simulink model "QuarterCarSim"  (R2026a)
settings: Solver=ode45  StopTime=5  RelTol=1e-8
undefined symbols (not defined in the file or in its folder): Amp, b_s, b_u, k_s, k_u, m_s, m_u, omega
settings Model: Creator=tyres  LastModifiedBy=tyres

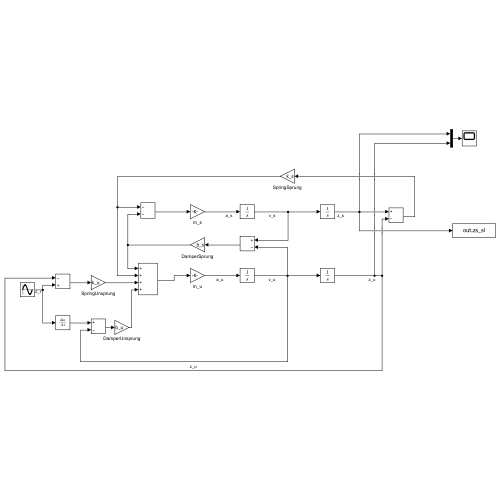
[thumbnail: Simulink's stored preview of the top-level diagram]
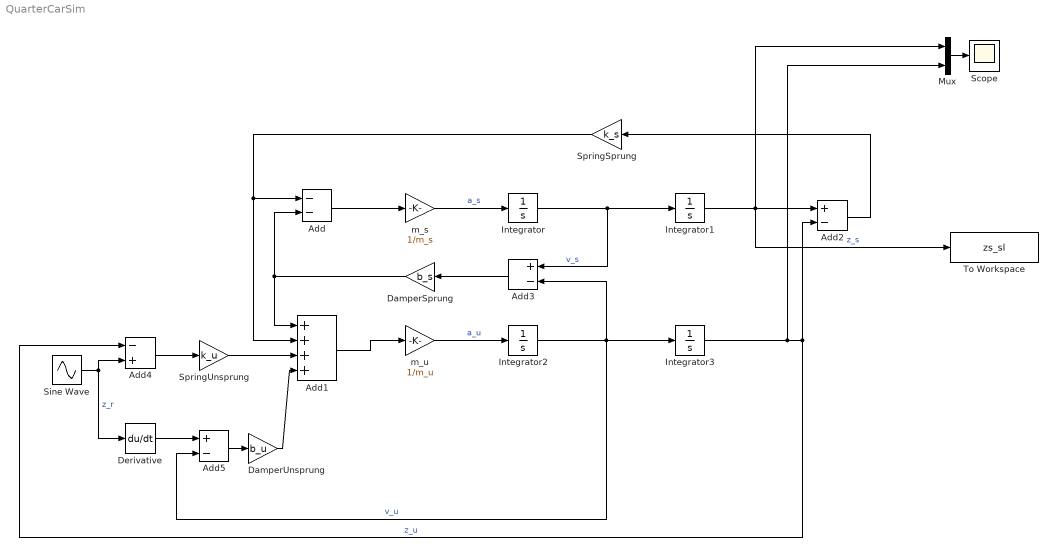
== system QuarterCarSim ==
  Add : Sum  Inputs=--
  Add1 : Sum  Inputs=++++
  Add2 : Sum  Inputs=+-
  Add3 : Sum  Inputs=+-
  Add4 : Sum  Inputs=-+
  Add5 : Sum  Inputs=+-
  DamperSprung : Gain  Gain=b_s
  DamperUnsprung : Gain  Gain=b_u
  Derivative : Derivative
  Integrator{,1..3} (4 alike) : Integrator
  Mux : Mux  Inputs=2
  Scope : Scope
      settings: ActiveDisplayYMinimum=-0.0072983920205625117  ActiveDisplayYMaximum=0.0069875189139344419
  Sine Wave : Sin  Amplitude=Amp  Frequency=omega  SampleTime=0
  SpringSprung : Gain  Gain=k_s
  SpringUnsprung : Gain  Gain=k_u
  To Workspace : ToWorkspace  VariableName=zs_sl  SaveFormat=Timeseries  SampleTime=-1
  m_s : Gain  Gain=1/m_s
  m_u : Gain  Gain=1/m_u
  wires:
  Integrator/1 -> Add3/1, Integrator1/1  "v_s"
  Integrator2/1 -> Add5/2, Add3/2, Integrator3/1  "v_u"
  m_s/1 -> Integrator/1  "a_s"
  Integrator3/1 -> Mux/2, Add4/1, Add2/2  "z_u"
  m_u/1 -> Integrator2/1  "a_u"
  Add1/1 -> m_u/1
  Add/1 -> m_s/1
  Integrator1/1 -> To Workspace/1, Mux/1, Add2/1  "z_s"
  Add2/1 -> SpringSprung/1
  SpringSprung/1 -> Add/1, Add1/2
  Add3/1 -> DamperSprung/1
  DamperSprung/1 -> Add1/1, Add/2
  Add4/1 -> SpringUnsprung/1
  SpringUnsprung/1 -> Add1/3
  Sine Wave/1 -> Derivative/1, Add4/2  "z_r"
  Derivative/1 -> Add5/1
  Add5/1 -> DamperUnsprung/1
  DamperUnsprung/1 -> Add1/4
  Mux/1 -> Scope/1
